simulink model "lab2_2"  (R2023a)
settings: Solver=VariableStepAuto  StartTime=0.0  StopTime=10  RelTol=1e-3
undefined symbols (not defined in the file or in its folder): K, x0
settings Model: Creator=bz  LastModifiedBy=bz

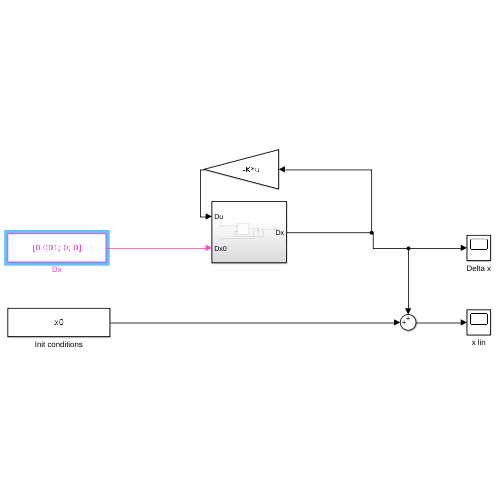
[thumbnail: Simulink's stored preview of the top-level diagram]
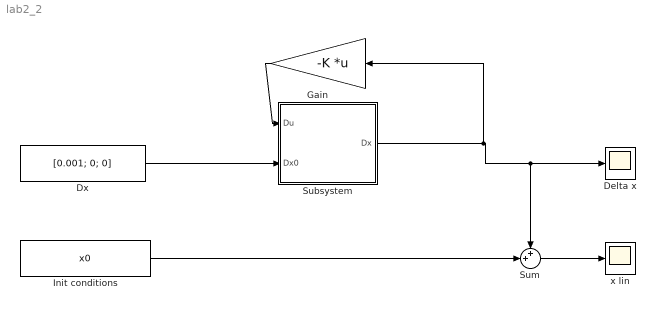
== system lab2_2 ==
  Delta x : Scope
  Dx : Constant  Value=[0.001; 0; 0]  VectorParams1D=off
  Gain : Gain  Gain=-K  Multiplication=Matrix(K*u)
  Init conditions : Constant  Value=x0  VectorParams1D=off
  Subsystem : Subsystem
  Sum : Sum  Inputs=++|
  x lin : Scope
  wires:
  Gain/1 -> Subsystem/1(Du)
  Dx/1 -> Subsystem/2(Dx0)
  Init conditions/1 -> Sum/2
  Subsystem/1(Dx) -> Gain/1, Sum/1, Delta x/1
  Sum/1 -> x lin/1

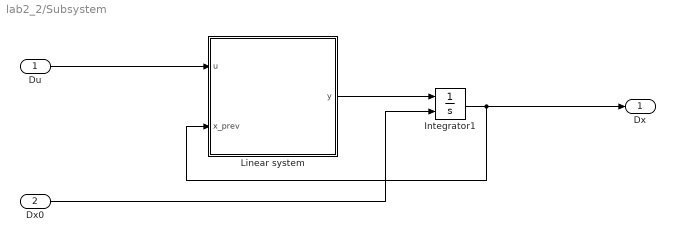
== system lab2_2/Subsystem ==
  Du : Inport
  Dx0 : Inport  Port=2
  Integrator1 : Integrator  InitialConditionSource=external
  Linear system : MATLAB Function  TreatAsAtomicUnit=on
  Dx : Outport
  wires:
  Linear system/1(y) -> Integrator1/1
  Dx0/1 -> Integrator1/2
  Integrator1/1 -> Dx/1, Linear system/2(x_prev)
  Du/1 -> Linear system/1(u)

== matlab function lab2_2/Subsystem/Linear system ==
  data: u input; y output size=[3,1]; x_prev input
function y  = fcn(u, x_prev)

A = [0              0.0010      0;
     1.6847         0           -0.0257;
     0              0           -0.2888] * 1e3;

B = [0;
     0;
     1.2706] * 1e3;

y = A * x_prev + B * u;

end
